simulink subsystem "MFTiresLongitudinal"  (R2023a)
settings: Solver=VariableStepAuto  StartTime=0.0  StopTime=10.0  RelTol=1e-3
libraries: autolibutils x2, autolibshared x2, autolibpowerinfoutils x2
(part 2 of 2)

== system MFTiresLongitudinal/Longitudinal Wheel - Front 2 ==
  Info : Inport
  Bus Selector : BusSelector  OutputSignals=PwrInfo.PwrTrnsfrd,PwrInfo.PwrNotTrnsfrd,PwrInfo.PwrStored
  Power Accounting Bus Creator : autolibpowerinfoutils/Power Accounting Bus Creator  AssctBlkSelPopup=Parent  RefBlkName='libraryname/blkname'  PwrTrnsfrdCheckBox=on  PwrNotTrnsfrdCheckBox=on  PwrStoredCheckBox=on  aMode=6
      settings: SourceProductName=Powertrain Blockset
  Terminator3 : Terminator
  wires:
  Power Accounting Bus Creator/1 -> Terminator3/1
  Bus Selector/3 -> Power Accounting Bus Creator/3  "<PwrStored>"
  Bus Selector/2 -> Power Accounting Bus Creator/2  "<PwrNotTrnsfrd>"
  Bus Selector/1 -> Power Accounting Bus Creator/1  "<PwrTrnsfrd>"
  Info/1 -> Bus Selector/1

== system MFTiresLongitudinal/Longitudinal Wheel - Rear 2 ==
  Info : Inport
  Bus Selector : BusSelector  OutputSignals=PwrInfo.PwrTrnsfrd,PwrInfo.PwrNotTrnsfrd,PwrInfo.PwrStored
  Power Accounting Bus Creator : autolibpowerinfoutils/Power Accounting Bus Creator  AssctBlkSelPopup=Parent  RefBlkName='libraryname/blkname'  PwrTrnsfrdCheckBox=on  PwrNotTrnsfrdCheckBox=on  PwrStoredCheckBox=on  aMode=6
      settings: SourceProductName=Powertrain Blockset
  Terminator3 : Terminator
  wires:
  Power Accounting Bus Creator/1 -> Terminator3/1
  Bus Selector/3 -> Power Accounting Bus Creator/3  "<PwrStored>"
  Bus Selector/2 -> Power Accounting Bus Creator/2  "<PwrNotTrnsfrd>"
  Bus Selector/1 -> Power Accounting Bus Creator/1  "<PwrTrnsfrd>"
  Info/1 -> Bus Selector/1

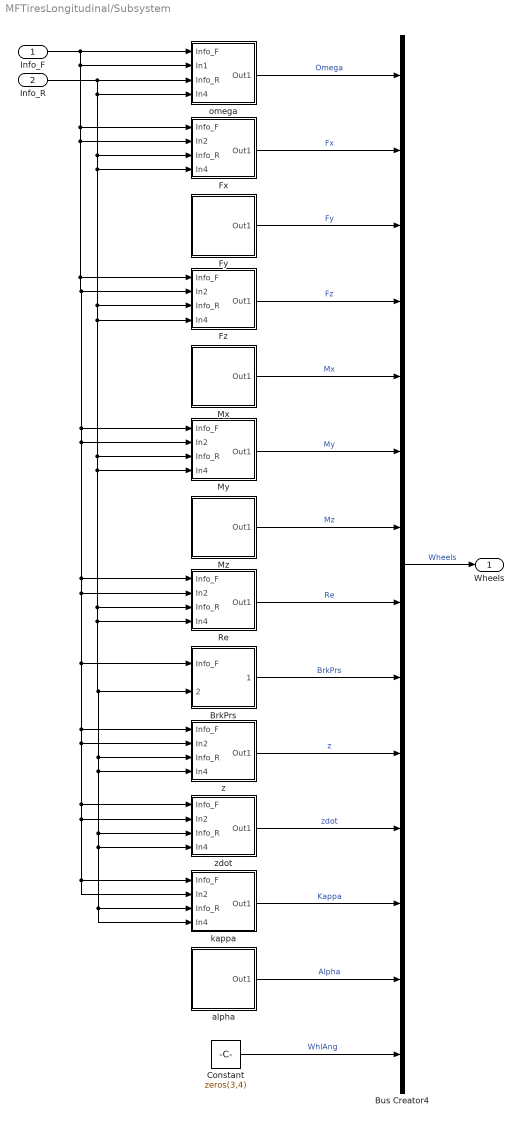
== system MFTiresLongitudinal/Subsystem ==
  Info_F : Inport
  Info_R : Inport  Port=2
  BrkPrs : Subsystem
  Bus Creator4 : BusCreator  Inputs=14
  Constant : Constant  Value=zeros(3,4)
  Fx : Subsystem
  Fy : Subsystem
  Fz : Subsystem
  Mx : Subsystem
  My : Subsystem
  Mz : Subsystem
  Re : Subsystem
  alpha : Subsystem
  kappa : Subsystem
  omega : Subsystem
  z : Subsystem
  zdot : Subsystem
  Wheels : Outport
  wires:
  Re/1(Out1) -> Bus Creator4/8  "Re"
  Fz/1(Out1) -> Bus Creator4/4  "Fz"
  Info_F/1 -> omega/2(In1), Fx/1(Info_F), Fx/2(In2), BrkPrs/1(Info_F), zdot/1(Info_F), kappa/1(Info_F), kappa/2(In2), zdot/2(In2), z/2(In2), z/1(Info_F), Re/2(In2), Re/1(Info_F), My/2(In2), My/1(Info_F), Fz/2(In2), Fz/1(Info_F), omega/1(Info_F)
  Info_R/1 -> Re/4(In4), BrkPrs/2(Info_R), kappa/3(Info_R), kappa/4(In4), zdot/4(In4), zdot/3(Info_R), z/4(In4), z/3(Info_R), Re/3(Info_R), My/4(In4), My/3(Info_R), Fz/4(In4), Fz/3(Info_R), Fx/4(In4), Fx/3(Info_R), omega/4(In4), omega/3(Info_R)
  Fx/1(Out1) -> Bus Creator4/2  "Fx"
  Mx/1(Out1) -> Bus Creator4/5  "Mx"
  zdot/1(Out1) -> Bus Creator4/11  "zdot"
  kappa/1(Out1) -> Bus Creator4/12  "Kappa"
  Mz/1(Out1) -> Bus Creator4/7  "Mz"
  omega/1(Out1) -> Bus Creator4/1  "Omega"
  z/1(Out1) -> Bus Creator4/10  "z"
  Fy/1(Out1) -> Bus Creator4/3  "Fy"
  My/1(Out1) -> Bus Creator4/6  "My"
  alpha/1(Out1) -> Bus Creator4/13  "Alpha"
  Bus Creator4/1 -> Wheels/1  "Wheels"
  BrkPrs/1(BrkPrs) -> Bus Creator4/9  "BrkPrs"
  Constant/1 -> Bus Creator4/14  "WhlAng"

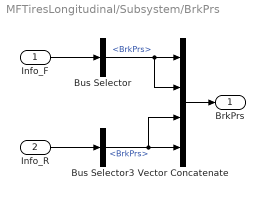
== system MFTiresLongitudinal/Subsystem/BrkPrs ==
  Info_F : Inport
  Info_R : Inport  Port=2
  Bus Selector : BusSelector  OutputSignals=BrkPrs
  Bus Selector3 : BusSelector  OutputSignals=BrkPrs
  Vector Concatenate : Concatenate  NumInputs=4
  BrkPrs : Outport  PortDimensions=4  VectorParamsAs1DForOutWhenUnconnected=off
  wires:
  Bus Selector/1 -> Vector Concatenate/2, Vector Concatenate/1  "<BrkPrs>"
  Info_F/1 -> Bus Selector/1
  Info_R/1 -> Bus Selector3/1
  Vector Concatenate/1 -> BrkPrs/1
  Bus Selector3/1 -> Vector Concatenate/3, Vector Concatenate/4  "<BrkPrs>"

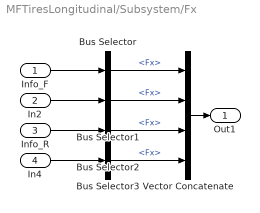
== system MFTiresLongitudinal/Subsystem/Fx ==
  Info_F : Inport
  In2 : Inport  Port=2
  Info_R : Inport  Port=3
  In4 : Inport  Port=4
  Bus Selector{,1..3} (4 alike) : BusSelector  OutputSignals=Fx
  Vector Concatenate : Concatenate  NumInputs=4
  Out1 : Outport  PortDimensions=4  VectorParamsAs1DForOutWhenUnconnected=off
  wires:
  Vector Concatenate/1 -> Out1/1
  Info_F/1 -> Bus Selector/1
  Bus Selector/1 -> Vector Concatenate/1  "<Fx>"
  In2/1 -> Bus Selector1/1
  Info_R/1 -> Bus Selector2/1
  In4/1 -> Bus Selector3/1
  Bus Selector1/1 -> Vector Concatenate/2  "<Fx>"
  Bus Selector2/1 -> Vector Concatenate/3  "<Fx>"
  Bus Selector3/1 -> Vector Concatenate/4  "<Fx>"

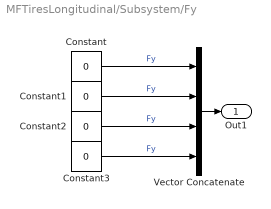
== system MFTiresLongitudinal/Subsystem/Fy ==
  Constant{,1..3} (4 alike) : Constant  Value=0  SampleTime=-1
  Vector Concatenate : Concatenate  NumInputs=4
  Out1 : Outport  PortDimensions=4  VectorParamsAs1DForOutWhenUnconnected=off
  wires:
  Constant/1 -> Vector Concatenate/1  "Fy"
  Vector Concatenate/1 -> Out1/1
  Constant1/1 -> Vector Concatenate/2  "Fy"
  Constant2/1 -> Vector Concatenate/3  "Fy"
  Constant3/1 -> Vector Concatenate/4  "Fy"

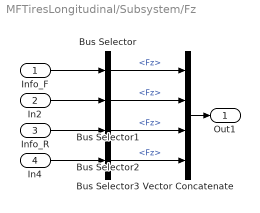
== system MFTiresLongitudinal/Subsystem/Fz ==
  Info_F : Inport
  In2 : Inport  Port=2
  Info_R : Inport  Port=3
  In4 : Inport  Port=4
  Bus Selector{,1..3} (4 alike) : BusSelector  OutputSignals=Fz
  Vector Concatenate : Concatenate  NumInputs=4
  Out1 : Outport  PortDimensions=4  VectorParamsAs1DForOutWhenUnconnected=off
  wires:
  Bus Selector3/1 -> Vector Concatenate/4  "<Fz>"
  Bus Selector2/1 -> Vector Concatenate/3  "<Fz>"
  Bus Selector1/1 -> Vector Concatenate/2  "<Fz>"
  In4/1 -> Bus Selector3/1
  Info_R/1 -> Bus Selector2/1
  In2/1 -> Bus Selector1/1
  Bus Selector/1 -> Vector Concatenate/1  "<Fz>"
  Info_F/1 -> Bus Selector/1
  Vector Concatenate/1 -> Out1/1

== system MFTiresLongitudinal/Subsystem/Mx ==
  Constant{,1..3} (4 alike) : Constant  Value=0  SampleTime=-1
  Vector Concatenate : Concatenate  NumInputs=4
  Out1 : Outport  PortDimensions=4  VectorParamsAs1DForOutWhenUnconnected=off
  wires:
  Vector Concatenate/1 -> Out1/1
  Constant1/1 -> Vector Concatenate/2  "Mx"
  Constant/1 -> Vector Concatenate/1  "Mx"
  Constant3/1 -> Vector Concatenate/4  "Mx"
  Constant2/1 -> Vector Concatenate/3  "Mx"

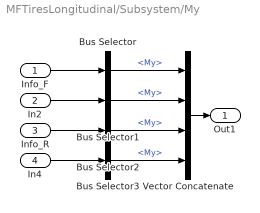
== system MFTiresLongitudinal/Subsystem/My ==
  Info_F : Inport
  In2 : Inport  Port=2
  Info_R : Inport  Port=3
  In4 : Inport  Port=4
  Bus Selector{,1..3} (4 alike) : BusSelector  OutputSignals=My
  Vector Concatenate : Concatenate  NumInputs=4
  Out1 : Outport  PortDimensions=4  VectorParamsAs1DForOutWhenUnconnected=off
  wires:
  Vector Concatenate/1 -> Out1/1
  Info_F/1 -> Bus Selector/1
  Bus Selector/1 -> Vector Concatenate/1  "<My>"
  In2/1 -> Bus Selector1/1
  Info_R/1 -> Bus Selector2/1
  In4/1 -> Bus Selector3/1
  Bus Selector1/1 -> Vector Concatenate/2  "<My>"
  Bus Selector2/1 -> Vector Concatenate/3  "<My>"
  Bus Selector3/1 -> Vector Concatenate/4  "<My>"

== system MFTiresLongitudinal/Subsystem/Mz ==
  Constant{,1..3} (4 alike) : Constant  Value=0  SampleTime=-1
  Vector Concatenate : Concatenate  NumInputs=4
  Out1 : Outport  PortDimensions=4  VectorParamsAs1DForOutWhenUnconnected=off
  wires:
  Vector Concatenate/1 -> Out1/1
  Constant1/1 -> Vector Concatenate/2  "Mz"
  Constant/1 -> Vector Concatenate/1  "Mz"
  Constant3/1 -> Vector Concatenate/4  "Mz"
  Constant2/1 -> Vector Concatenate/3  "Mz"

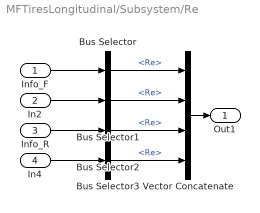
== system MFTiresLongitudinal/Subsystem/Re ==
  Info_F : Inport
  In2 : Inport  Port=2
  Info_R : Inport  Port=3
  In4 : Inport  Port=4
  Bus Selector{,1..3} (4 alike) : BusSelector  OutputSignals=Re
  Vector Concatenate : Concatenate  NumInputs=4
  Out1 : Outport  PortDimensions=4  VectorParamsAs1DForOutWhenUnconnected=off
  wires:
  Bus Selector3/1 -> Vector Concatenate/4  "<Re>"
  Bus Selector2/1 -> Vector Concatenate/3  "<Re>"
  Bus Selector1/1 -> Vector Concatenate/2  "<Re>"
  In4/1 -> Bus Selector3/1
  Info_R/1 -> Bus Selector2/1
  In2/1 -> Bus Selector1/1
  Bus Selector/1 -> Vector Concatenate/1  "<Re>"
  Info_F/1 -> Bus Selector/1
  Vector Concatenate/1 -> Out1/1

== system MFTiresLongitudinal/Subsystem/alpha ==
  Constant{,1..3} (4 alike) : Constant  Value=0  SampleTime=-1
  Vector Concatenate : Concatenate  NumInputs=4
  Out1 : Outport  PortDimensions=4  VectorParamsAs1DForOutWhenUnconnected=off
  wires:
  Vector Concatenate/1 -> Out1/1
  Constant1/1 -> Vector Concatenate/2  "Alpha"
  Constant/1 -> Vector Concatenate/1  "Alpha"
  Constant3/1 -> Vector Concatenate/4  "Alpha"
  Constant2/1 -> Vector Concatenate/3  "Alpha"

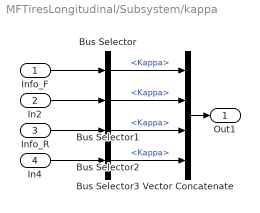
== system MFTiresLongitudinal/Subsystem/kappa ==
  Info_F : Inport
  In2 : Inport  Port=2
  Info_R : Inport  Port=3
  In4 : Inport  Port=4
  Bus Selector{,1..3} (4 alike) : BusSelector  OutputSignals=Kappa
  Vector Concatenate : Concatenate  NumInputs=4
  Out1 : Outport  PortDimensions=4  VectorParamsAs1DForOutWhenUnconnected=off
  wires:
  Vector Concatenate/1 -> Out1/1
  Info_F/1 -> Bus Selector/1
  Bus Selector/1 -> Vector Concatenate/1  "<Kappa>"
  In2/1 -> Bus Selector1/1
  Info_R/1 -> Bus Selector2/1
  In4/1 -> Bus Selector3/1
  Bus Selector1/1 -> Vector Concatenate/2  "<Kappa>"
  Bus Selector2/1 -> Vector Concatenate/3  "<Kappa>"
  Bus Selector3/1 -> Vector Concatenate/4  "<Kappa>"

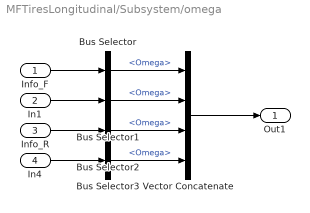
== system MFTiresLongitudinal/Subsystem/omega ==
  Info_F : Inport
  In1 : Inport  Port=2
  Info_R : Inport  Port=3
  In4 : Inport  Port=4
  Bus Selector{,1..3} (4 alike) : BusSelector  OutputSignals=Omega
  Vector Concatenate : Concatenate  NumInputs=4
  Out1 : Outport  PortDimensions=4  VectorParamsAs1DForOutWhenUnconnected=off
  wires:
  Vector Concatenate/1 -> Out1/1
  Bus Selector3/1 -> Vector Concatenate/4  "<Omega>"
  Bus Selector2/1 -> Vector Concatenate/3  "<Omega>"
  Bus Selector1/1 -> Vector Concatenate/2  "<Omega>"
  In4/1 -> Bus Selector3/1
  Info_R/1 -> Bus Selector2/1
  In1/1 -> Bus Selector1/1
  Bus Selector/1 -> Vector Concatenate/1  "<Omega>"
  Info_F/1 -> Bus Selector/1

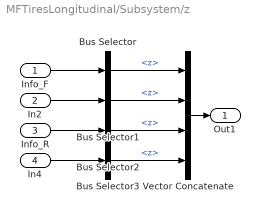
== system MFTiresLongitudinal/Subsystem/z ==
  Info_F : Inport
  In2 : Inport  Port=2
  Info_R : Inport  Port=3
  In4 : Inport  Port=4
  Bus Selector{,1..3} (4 alike) : BusSelector  OutputSignals=z
  Vector Concatenate : Concatenate  NumInputs=4
  Out1 : Outport  PortDimensions=4  VectorParamsAs1DForOutWhenUnconnected=off
  wires:
  Vector Concatenate/1 -> Out1/1
  Info_F/1 -> Bus Selector/1
  Bus Selector/1 -> Vector Concatenate/1  "<z>"
  In2/1 -> Bus Selector1/1
  Info_R/1 -> Bus Selector2/1
  In4/1 -> Bus Selector3/1
  Bus Selector1/1 -> Vector Concatenate/2  "<z>"
  Bus Selector2/1 -> Vector Concatenate/3  "<z>"
  Bus Selector3/1 -> Vector Concatenate/4  "<z>"

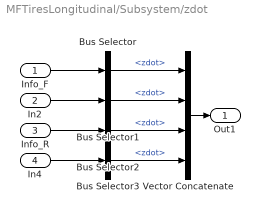
== system MFTiresLongitudinal/Subsystem/zdot ==
  Info_F : Inport
  In2 : Inport  Port=2
  Info_R : Inport  Port=3
  In4 : Inport  Port=4
  Bus Selector{,1..3} (4 alike) : BusSelector  OutputSignals=zdot
  Vector Concatenate : Concatenate  NumInputs=4
  Out1 : Outport  PortDimensions=4  VectorParamsAs1DForOutWhenUnconnected=off
  wires:
  Bus Selector3/1 -> Vector Concatenate/4  "<zdot>"
  Bus Selector2/1 -> Vector Concatenate/3  "<zdot>"
  Bus Selector1/1 -> Vector Concatenate/2  "<zdot>"
  In4/1 -> Bus Selector3/1
  Info_R/1 -> Bus Selector2/1
  In2/1 -> Bus Selector1/1
  Bus Selector/1 -> Vector Concatenate/1  "<zdot>"
  Info_F/1 -> Bus Selector/1
  Vector Concatenate/1 -> Out1/1
